simulink model "atividade_04_exemplo"  (R2024b)
settings: Solver=VariableStepAuto  StartTime=0.0  StopTime=10.0  RelTol=1e-3
libraries: slpidlib x4
settings Model: Creator=victo

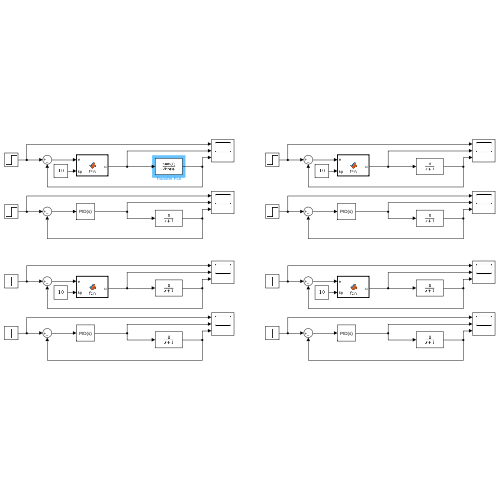
[thumbnail: Simulink's stored preview of the top-level diagram]
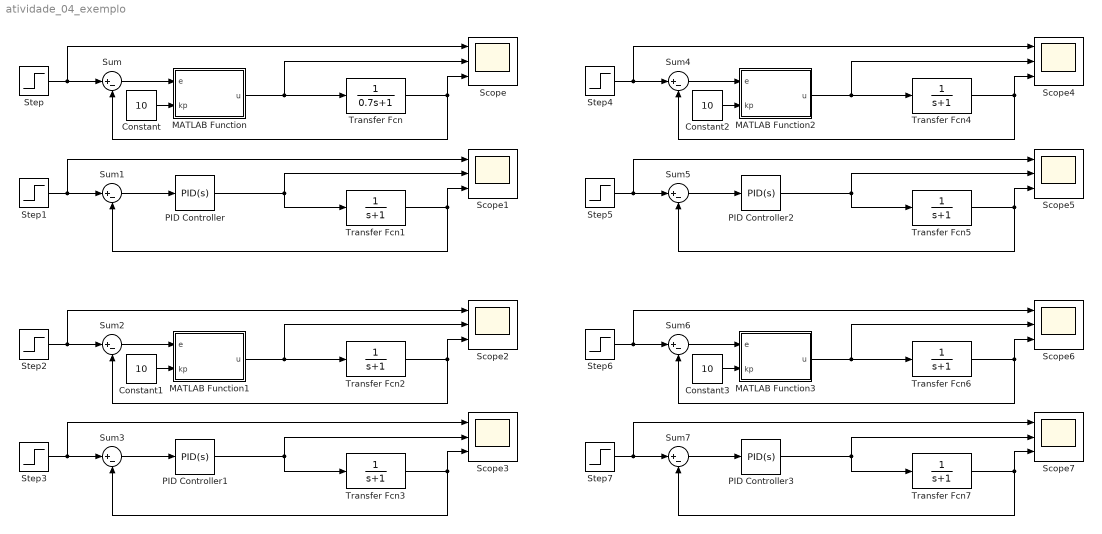
== system atividade_04_exemplo ==
  Constant{,1..3} (4 alike) : Constant  Value=10
  MATLAB Function : MATLAB Function  TreatAsAtomicUnit=on
  MATLAB Function1 : MATLAB Function  TreatAsAtomicUnit=on
  MATLAB Function2 : MATLAB Function  TreatAsAtomicUnit=on
  MATLAB Function3 : MATLAB Function  TreatAsAtomicUnit=on
  PID Controller{,1..3} (4 alike) : slpidlib/PID Controller  Controller=PID  Form=Parallel  TimeDomain=Continuous-time  UseExternalTs=off  SampleTime=-1  IntegratorMethod=Forward Euler  FilterMethod=Forward Euler  ControllerParametersSource=internal  P=10  I=0  UseKiTs=off  D=0  UseExternalDerivativeSource=off  N=100  UseFilter=on  TunerSelectOption=Transfer Function Based (PID Tuner App)  InitialConditionSource=internal  InitialConditionForIntegrator=0  InitialConditionForFilter=0  DifferentiatorICPrevScaledInput=0  ExternalReset=none  TrackingMode=off  Kt=1  LimitOutput=off  SatLimitsSource=internal  UpperSaturationLimit=inf  LowerSaturationLimit=-inf  LinearizeAsGain=on  AntiWindupMode=none  Kb=1  LimitIntegrator=off  UpperIntegratorSaturationLimit=inf  LowerIntegratorSaturationLimit=-inf  POutMin=[]  POutMax=[]  IOutMin=[]  IOutMax=[]  DOutMin=[]  DOutMax=[]  NOutMin=[]  NOutMax=[]  SumOutMin=[]  SumOutMax=[]  SaturationOutMin=[]  SaturationOutMax=[]  PParamMin=[]  PParamMax=[]  IParamMin=[]  IParamMax=[]  DParamMin=[]  DParamMax=[]  NParamMin=[]  NParamMax=[]  KbParamMin=[]  KbParamMax=[]  KtParamMin=[]  KtParamMax=[]  KbOutMin=[]  KbOutMax=[]  KtOutMin=[]  KtOutMax=[]  IntegratorOutMin=[]  IntegratorOutMax=[]  FilterOutMin=[]  FilterOutMax=[]  SumI1OutMin=[]  SumI1OutMax=[]  SumI2OutMin=[]  SumI2OutMax=[]  SumI3OutMin=[]  SumI3OutMax=[]  SumI4OutMin=[]  SumI4OutMax=[]  SumDOutMin=[]  SumDOutMax=[]  DifferentiatorOutMin=[]  DifferentiatorOutMax=[]  FilterDiffOutCoefMin=[]  FilterDiffOutCoefMax=[]  ReciprocalOutMin=[]  ReciprocalOutMax=[]  SumDenOutMin=[]  SumDenOutMax=[]  SumNumOutMin=[]  SumNumOutMax=[]  DivideOutMin=[]  DivideOutMax=[]  UdiffTsProdOutMin=[]  UdiffTsProdOutMax=[]  NTsProdOutMin=[]  NTsProdOutMax=[]  UintegralTsProdOutMin=[]  UintegralTsProdOutMax=[]  UngainTsProdOutMin=[]  UngainTsProdOutMax=[]  ClampingZeroOutDataTypeStr=Inherit: Inherit via back propagation  ClampingZeroOutMin=[]  ClampingZeroOutMax=[]  FilterDenConstantOutDataTypeStr=Inherit: Inherit via back propagation  FilterDenConstantOutMin=[]  FilterDenConstantOutMax=[]  PCopyOutDataTypeStr=Inherit: Inherit via back propagation  PCopyOutMin=[]  PCopyOutMax=[]  NCopyOutDataTypeStr=Inherit: Inherit via back propagation  NCopyOutMin=[]  NCopyOutMax=[]  IntegratorContinuousStateAttributes=''  IntegratorStateMustResolveToSignalObject=off  IntegratorRTWStateStorageClass=Auto  FilterContinuousStateAttributes=''  FilterStateMustResolveToSignalObject=off  FilterRTWStateStorageClass=Auto  ParallelPVariant=InternalParameters  IdealPVariant=Disabled  IVariant=InternalParameters  DVariant=InternalParameters  IntegratorVariant=Continuous  SatVariant=Disabled  AWVariant=Passthrough  PCopyVariant=Disabled  TRVariant=Disabled  FdbkBlocksVariant=Forward  IdealPFdbkVariant=Disabled  SatFdbkVariant=Disabled  DerivativeFilterVariant=ContFilter  NVariant=InternalParameters  NCopyVariant=Disabled  FilterICVariant=InternalICsFilter  IntegratorICVariant=InternalICs  ExternalResetVariant=Disabled  TRSumVariant=Passthrough  SumFdbkVariant=Disabled  SumVariant=Sum_PID  TsampFilterVariant=InternalTs  TsampNgainVariant=Passthrough  TsampIntegralVariant=Disabled_SignalSpec  ExternalSaturationOutDataTypeStr=Inherit: Same as second input  DerivativeSourceVariant=ErrorSignal  PreIntVariant=InternalPreInt
  Scope{,1..7} (8 alike) : Scope  NumInputPorts=3
  Step{,1..7} (8 alike) : Step  SampleTime=0
  Sum{,1..7} (8 alike) : Sum  Inputs=|+-
  Transfer Fcn : TransferFcn  Denominator=[0.7 1]
  Transfer Fcn{1..7} (7 alike) : TransferFcn  Denominator=[1 1]
  wires:
  Step/1 -> Scope/1, Sum/1
  Sum/1 -> MATLAB Function/1(e)
  MATLAB Function/1(u) -> Scope/2, Transfer Fcn/1
  Transfer Fcn/1 -> Scope/3, Sum/2
  Constant/1 -> MATLAB Function/2(kp)
  Transfer Fcn1/1 -> Scope1/3, Sum1/2
  Sum1/1 -> PID Controller/1
  Step1/1 -> Scope1/1, Sum1/1
  PID Controller/1 -> Transfer Fcn1/1, Scope1/2
  Transfer Fcn3/1 -> Scope3/3, Sum3/2
  Transfer Fcn2/1 -> Scope2/3, Sum2/2
  Sum3/1 -> PID Controller1/1
  Constant1/1 -> MATLAB Function1/2(kp)
  MATLAB Function1/1(u) -> Scope2/2, Transfer Fcn2/1
  PID Controller1/1 -> Transfer Fcn3/1, Scope3/2
  Sum2/1 -> MATLAB Function1/1(e)
  Step3/1 -> Scope3/1, Sum3/1
  Step2/1 -> Scope2/1, Sum2/1
  Transfer Fcn5/1 -> Scope5/3, Sum5/2
  Transfer Fcn4/1 -> Scope4/3, Sum4/2
  Sum5/1 -> PID Controller2/1
  Constant2/1 -> MATLAB Function2/2(kp)
  MATLAB Function2/1(u) -> Scope4/2, Transfer Fcn4/1
  PID Controller2/1 -> Transfer Fcn5/1, Scope5/2
  Sum4/1 -> MATLAB Function2/1(e)
  Step5/1 -> Scope5/1, Sum5/1
  Step4/1 -> Scope4/1, Sum4/1
  Transfer Fcn7/1 -> Scope7/3, Sum7/2
  Transfer Fcn6/1 -> Scope6/3, Sum6/2
  Sum7/1 -> PID Controller3/1
  Constant3/1 -> MATLAB Function3/2(kp)
  MATLAB Function3/1(u) -> Scope6/2, Transfer Fcn6/1
  PID Controller3/1 -> Transfer Fcn7/1, Scope7/2
  Sum6/1 -> MATLAB Function3/1(e)
  Step7/1 -> Scope7/1, Sum7/1
  Step6/1 -> Scope6/1, Sum6/1

== matlab function atividade_04_exemplo/MATLAB Function ==
  data: e input; u output; kp input
function u = fcn(e, kp)

u = kp*e;

== matlab function atividade_04_exemplo/MATLAB Function2 ==
  data: e input; u output; kp input
function u = fcn(e, kp)

u = kp*e;

== matlab function atividade_04_exemplo/MATLAB Function3 ==
  data: e input; u output; kp input
function u = fcn(e, kp)

u = kp*e;

== matlab function atividade_04_exemplo/MATLAB Function1 ==
  data: e input; u output; kp input
function u = fcn(e, kp)

u = kp*e;
